simulink model "feature2_cc_automate"  (R2020b)
settings: Solver=VariableStepAuto  StartTime=0.0  StopTime=inf  RelTol=1e-3
settings Model: Creator=99003757  LastModifiedBy=99003757

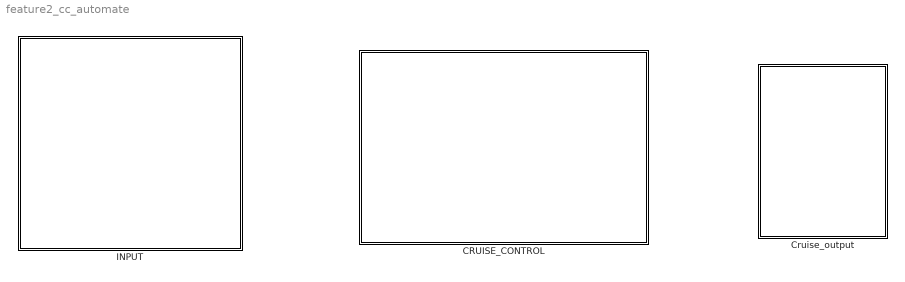
== system feature2_cc_automate ==
  CRUISE_CONTROL : Subsystem
  Cruise_output : Subsystem
  INPUT : Subsystem

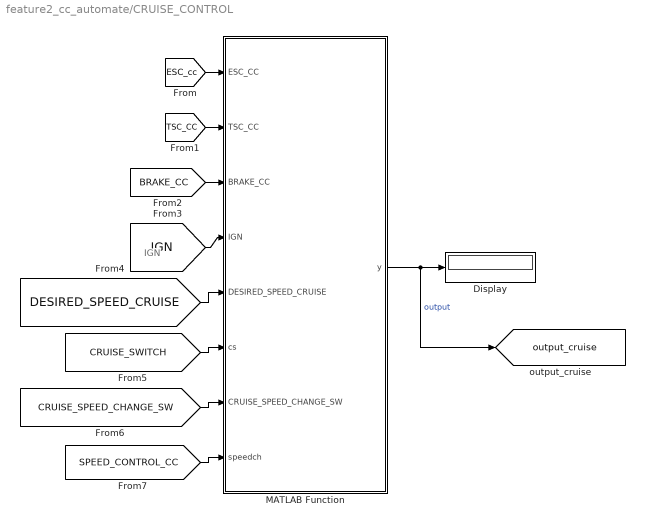
== system feature2_cc_automate/CRUISE_CONTROL ==
  note: IGN
  Display : Display
  MATLAB Function : MATLAB Function  TreatAsAtomicUnit=on
  tag scope: output_cruise=global
  wires:
  [DESIRED_SPEED_CRUISE] -> MATLAB Function/5(DESIRED_SPEED_CRUISE)
  [BRAKE_CC] -> MATLAB Function/3(BRAKE_CC)
  [CRUISE_SWITCH] -> MATLAB Function/6(cs)
  [ESC_cc] -> MATLAB Function/1(ESC_CC)
  [SPEED_CONTROL_CC] -> MATLAB Function/8(speedch)
  MATLAB Function/1(y) -> [output_cruise], Display/1  "output"
  [TSC_CC] -> MATLAB Function/2(TSC_CC)
  [IGN] -> MATLAB Function/4(IGN)
  [CRUISE_SPEED_CHANGE_SW] -> MATLAB Function/7(CRUISE_SPEED_CHANGE_SW)

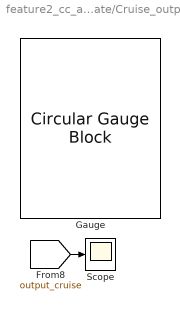
== system feature2_cc_automate/Cruise_output ==
  Gauge : CircularGaugeBlock
  Scope : Scope
  wires:
  [output_cruise] -> Scope/1

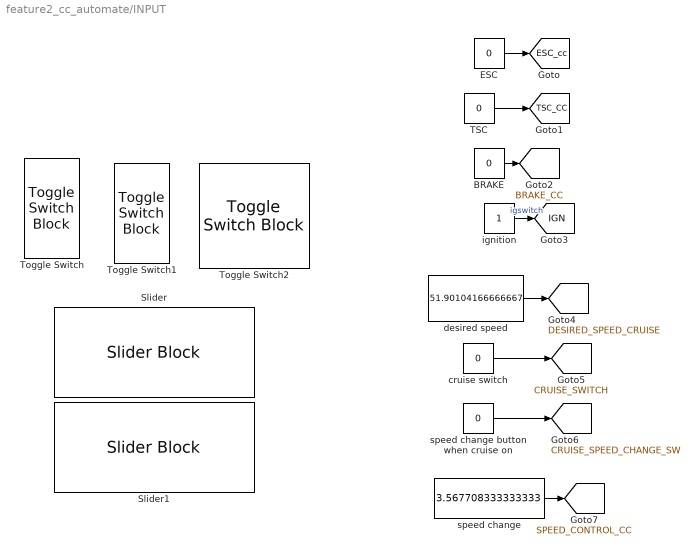
== system feature2_cc_automate/INPUT ==
  BRAKE : Constant  Value=0
  ESC : Constant  Value=0
  Slider : SliderBlock
  Slider1 : SliderBlock
  TSC : Constant  Value=0
  Toggle Switch : ToggleSwitchBlock
      settings: Values={{'Off', 'On'}, [0 1]}
  Toggle Switch1 : ToggleSwitchBlock
      settings: Values={{'Off', 'On'}, [0 1]}
  Toggle Switch2 : ToggleSwitchBlock
      settings: Values={{'Off', 'On'}, [0 1]}
  cruise switch : Constant  Value=0
  desired speed : Constant  Value=51.90104166666667
  "ignition " : Constant
  speed change : Constant  Value=3.567708333333333
  "speed change button when cruise on " : Constant  Value=0
  tag scope: BRAKE_CC=global, CRUISE_SPEED_CHANGE_SW=global, CRUISE_SWITCH=global, DESIRED_SPEED_CRUISE=global, ESC_cc=global, IGN=global, SPEED_CONTROL_CC=global, TSC_CC=global
  wires:
  "ignition "/1 -> [IGN]  "igswitch"
  cruise switch/1 -> [CRUISE_SWITCH]
  BRAKE/1 -> [BRAKE_CC]
  desired speed/1 -> [DESIRED_SPEED_CRUISE]
  "speed change button when cruise on "/1 -> [CRUISE_SPEED_CHANGE_SW]
  TSC/1 -> [TSC_CC]
  ESC/1 -> [ESC_cc]
  speed change/1 -> [SPEED_CONTROL_CC]

== matlab function feature2_cc_automate/CRUISE_CONTROL/MATLAB Function ==
  data: ESC_CC input; TSC_CC input; BRAKE_CC input; IGN input; y output; DESIRED_SPEED_CRUISE input; cs input; CRUISE_SPEED_CHANGE_SW input; speedch input
function y = fcn(ESC_CC, TSC_CC, BRAKE_CC, IGN, DESIRED_SPEED_CRUISE, cs, CRUISE_SPEED_CHANGE_SW, speedch)

if (IGN==1&& ESC_CC==0 &&TSC_CC==0 && BRAKE_CC==0)
    if (cs ==1 && DESIRED_SPEED_CRUISE>40 && CRUISE_SPEED_CHANGE_SW==1)
        y= DESIRED_SPEED_CRUISE+speedch;
    else
        y=DESIRED_SPEED_CRUISE;
    end
      
else
    y=0;
end
